simulink model "BPSKModulation"  (R2019b)
settings: Solver=VariableStepAuto  StartTime=0.0  StopTime=10.0  RelTol=1e-3
libraries: simulink x1
settings Model: Creator=z3454314  LastModifiedBy=z3454314

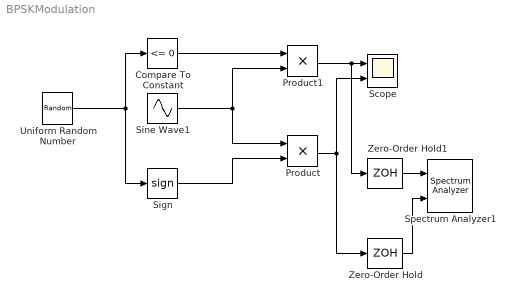
== system BPSKModulation ==
  Compare To Constant : simulink/Logic and Bit Operations/Compare To Constant  relop=<=  const=0  OutDataTypeStr=boolean
  Product : Product
  Product1 : Product
  Scope : Scope  NumInputPorts=2
  Sign : Signum
  Sine Wave1 : Sin  Frequency=8000*2*pi  SampleTime=0
  Spectrum Analyzer1 : SpectrumAnalyzer  NumInputPorts=2
  Uniform Random Number : UniformRandomNumber  SampleTime=1/500
  Zero-Order Hold : ZeroOrderHold  SampleTime=1/50000
  Zero-Order Hold1 : ZeroOrderHold  SampleTime=1/50000
  wires:
  Uniform Random Number/1 -> Compare To Constant/1, Sign/1
  Compare To Constant/1 -> Product1/1
  Sign/1 -> Product/2
  Sine Wave1/1 -> Product/1, Product1/2
  Product1/1 -> Zero-Order Hold1/1, Scope/1
  Product/1 -> Scope/2, Zero-Order Hold/1
  Zero-Order Hold/1 -> Spectrum Analyzer1/2
  Zero-Order Hold1/1 -> Spectrum Analyzer1/1
